simulink model "mysim"  (R2018b)
settings: Solver=VariableStepAuto  StartTime=0.0  StopTime=10.0  RelTol=1e-3
settings Model: Creator=12732  LastModifiedBy=12732

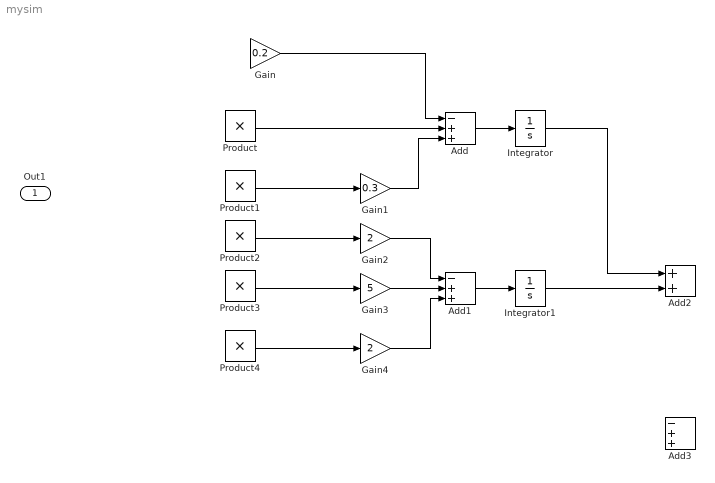
== system mysim ==
  Add : Sum  Inputs=-++
  Add1 : Sum  Inputs=-++
  Add2 : Sum
  Add3 : Sum  Inputs=-++
  Gain : Gain  Gain=0.2
  Gain1 : Gain  Gain=0.3
  Gain2 : Gain  Gain=2
  Gain3 : Gain  Gain=5
  Gain4 : Gain  Gain=2
  Integrator : Integrator  InitialCondition=0.8
  Integrator1 : Integrator  InitialCondition=0.8
  Product{,1..4} (5 alike) : Product
  Out1 : Outport
  wires:
  Gain/1 -> Add/1
  Product/1 -> Add/2
  Product1/1 -> Gain1/1
  Gain1/1 -> Add/3
  Product2/1 -> Gain2/1
  Product3/1 -> Gain3/1
  Product4/1 -> Gain4/1
  Gain2/1 -> Add1/1
  Gain3/1 -> Add1/2
  Gain4/1 -> Add1/3
  Add/1 -> Integrator/1
  Integrator/1 -> Add2/1
  Add1/1 -> Integrator1/1
  Integrator1/1 -> Add2/2
